simulink model "sistema_termico"  (R2016b)
settings: Solver=VariableStepAuto  StartTime=0.0  StopTime=10.0  RelTol=1e-3
values from neighbouring files (symbols this model uses):
  Cts = .818    (= 0.818)    [c4ModeloCompleto.m]    (also in c4ModeloCompleto_var.m)
  Rs = 1.02    [c4ModeloCompleto_var.m]
  Rts_amb = 146.7    [c4ModeloCompleto.m]    (also in c4ModeloCompleto_var.m)
settings Model: Creator=agustin  LastModifiedBy=agustin

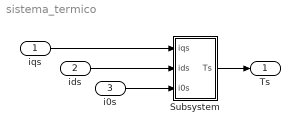
== system sistema_termico ==
  iqs : Inport
  ids : Inport  Port=2
  "i0s " : Inport  Port=3
  Subsystem : Subsystem
  Ts : Outport
  wires:
  iqs/1 -> Subsystem/1(iqs)
  ids/1 -> Subsystem/2(ids)
  "i0s "/1 -> Subsystem/3("i0s ")
  Subsystem/1(Ts) -> Ts/1

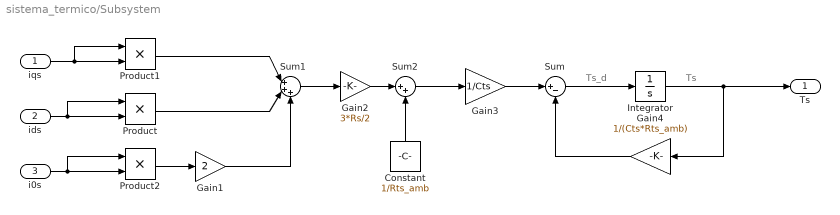
== system sistema_termico/Subsystem ==
  note: Ts_d
  note: Ts
  iqs : Inport
  ids : Inport  Port=2
  "i0s " : Inport  Port=3
  Constant : Constant  Value=1/Rts_amb
  Gain1 : Gain  Gain=2
  Gain2 : Gain  Gain=3*Rs/2
  Gain3 : Gain  Gain=1/Cts
  Gain4 : Gain  Gain=1/(Cts*Rts_amb)
  Integrator : Integrator
  Product : Product
  Product1 : Product
  Product2 : Product
  Sum : Sum  Inputs=|+-
  Sum1 : Sum  Inputs=|+++
  Sum2 : Sum  Inputs=|++
  Ts : Outport
  wires:
  iqs/1 -> Product1/1, Product1/2
  Gain2/1 -> Sum2/1
  Constant/1 -> Sum2/2
  Product1/1 -> Sum1/1
  Sum2/1 -> Gain3/1
  Gain3/1 -> Sum/1
  Sum/1 -> Integrator/1
  Product2/1 -> Gain1/1
  "i0s "/1 -> Product2/1, Product2/2
  ids/1 -> Product/1, Product/2
  Integrator/1 -> Ts/1, Gain4/1
  Product/1 -> Sum1/2
  Gain1/1 -> Sum1/3
  Sum1/1 -> Gain2/1
  Gain4/1 -> Sum/2
